simulink model "connect_fbk_R2018a"  (R2018a)
settings: Solver=VariableStepAuto  StartTime=0.0  StopTime=10.0  RelTol=1e-3
settings Model: Creator=kawata  LastModifiedBy=kawata

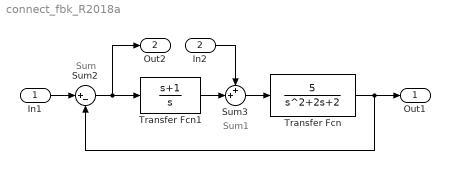
== system connect_fbk_R2018a ==
  note: Sum
  note: Sum1
  In1 : Inport
  In2 : Inport  Port=2
  Sum2 : Sum  Inputs=|+-
  Sum3 : Sum  Inputs=++|
  Transfer Fcn : TransferFcn  Numerator=[5]  Denominator=[1 2 2]
  Transfer Fcn1 : TransferFcn  Numerator=[1 1]  Denominator=[1 0]
  Out1 : Outport  VectorParamsAs1DForOutWhenUnconnected=off
  Out2 : Outport  Port=2  VectorParamsAs1DForOutWhenUnconnected=off
  wires:
  In1/1 -> Sum2/1
  In2/1 -> Sum3/1
  Transfer Fcn1/1 -> Sum3/2
  Transfer Fcn/1 -> Out1/1, Sum2/2
  Sum2/1 -> Transfer Fcn1/1, Out2/1
  Sum3/1 -> Transfer Fcn/1
